simulink model "runTrajectoryFuzzy"  (R2019a)
settings: Solver=ode3  StartTime=0.0  StopTime=100.0  FixedStep=Ts  RelTol=1e-3
undefined symbols (not defined in the file): DiscIntNeverNeededParam, sigbuilder_block, th_0, Ts, x_0, y_0
libraries: simulink x3, fuzblock x1
settings Model: Creator=alvar  LastModifiedBy=alvar

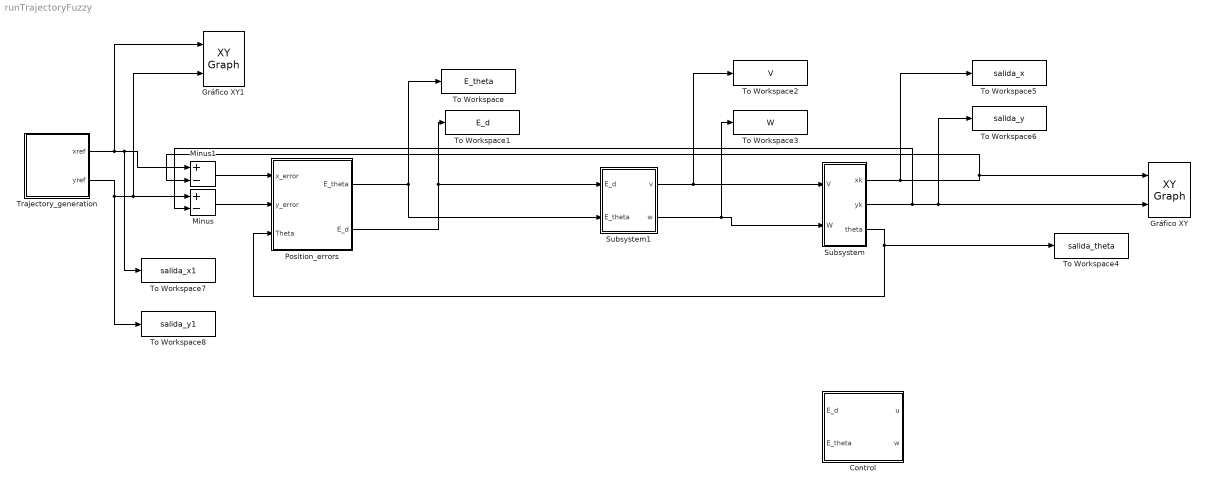
== system runTrajectoryFuzzy ==
  Control : Subsystem
  Gráfico XY : simulink/Sinks/XY Graph  xmin=-5  xmax=5  ymin=-5  ymax=5  st=-1
  Gráfico XY1 : simulink/Sinks/XY Graph  xmin=-5  xmax=5  ymin=-5  ymax=5  st=-1
  Minus : Sum  Inputs=+-
  Minus1 : Sum  Inputs=+-
  Position_errors : Subsystem
  Subsystem : Subsystem
  Subsystem1 : Subsystem
  To Workspace : ToWorkspace  VariableName=E_theta  SaveFormat=Structure With Time  SampleTime=-1
  To Workspace1 : ToWorkspace  VariableName=E_d  SaveFormat=Structure With Time  SampleTime=-1
  To Workspace2 : ToWorkspace  VariableName=V  SaveFormat=Structure With Time  SampleTime=-1
  To Workspace3 : ToWorkspace  VariableName=W  SaveFormat=Structure With Time  SampleTime=-1
  To Workspace4 : ToWorkspace  VariableName=salida_theta  SaveFormat=Structure With Time  SampleTime=-1
  To Workspace5 : ToWorkspace  VariableName=salida_x  SaveFormat=Structure With Time  SampleTime=-1
  To Workspace6 : ToWorkspace  VariableName=salida_y  SaveFormat=Structure With Time  SampleTime=-1
  To Workspace7 : ToWorkspace  VariableName=salida_x1  SaveFormat=Structure With Time  SampleTime=-1
  To Workspace8 : ToWorkspace  VariableName=salida_y1  SaveFormat=Structure With Time  SampleTime=-1
  Trajectory_generation : Subsystem
  wires:
  Position_errors/2(E_d) -> Subsystem1/1("E_d "), To Workspace1/1
  Subsystem1/1(v) -> To Workspace2/1, Subsystem/1(V)
  Minus/1 -> Position_errors/2("y_error ")
  Subsystem/1(xk) -> To Workspace5/1, Minus1/2, Gráfico XY/1
  Subsystem/3("theta ") -> Position_errors/3(Theta), To Workspace4/1
  Trajectory_generation/1(xref) -> Gráfico XY1/1, To Workspace7/1, Minus1/1
  Trajectory_generation/2(yref) -> To Workspace8/1, Gráfico XY1/2, Minus/1
  Subsystem/2(yk) -> Minus/2, To Workspace6/1, Gráfico XY/2
  Subsystem1/2(w) -> To Workspace3/1, Subsystem/2("W ")
  Position_errors/1(E_theta) -> Subsystem1/2(E_theta), To Workspace/1
  Minus1/1 -> Position_errors/1("x_error ")

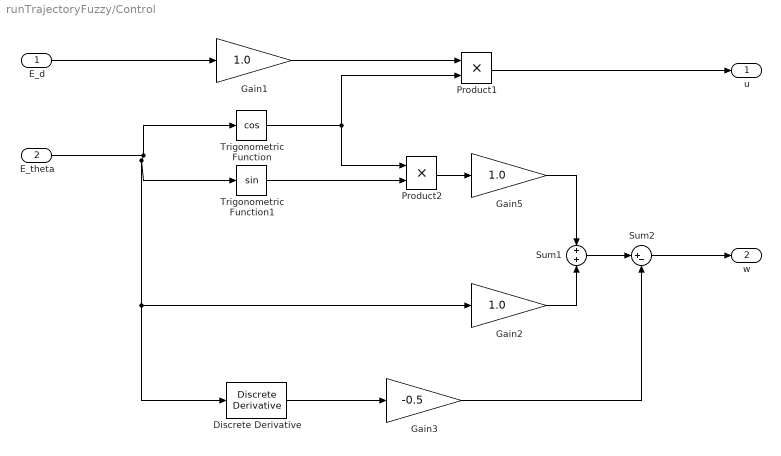
== system runTrajectoryFuzzy/Control ==
  E_d : Inport
  E_theta : Inport  Port=2
  Discrete Derivative : simulink/Discrete/Discrete Derivative  gainval=1.0  ICPrevScaledInput=0.0  OutMin=[]  OutMax=[]  OutDataType=fixdt(1, 16)  OutScaling=2^-10  DoSatur=off
  Gain1 : Gain  Gain=1.0
  Gain2 : Gain  Gain=1.0
  Gain3 : Gain  Gain=-0.5
  Gain5 : Gain  Gain=1.0
  Product1 : Product
  Product2 : Product
  Sum1 : Sum
  Sum2 : Sum  Inputs=|+-
  Trigonometric Function : Trigonometry  Operator=cos
  Trigonometric Function1 : Trigonometry
  u : Outport
  w : Outport  Port=2
  wires:
  E_theta/1 -> Trigonometric Function/1, Trigonometric Function1/1, Discrete Derivative/1, Gain2/1
  E_d/1 -> Gain1/1
  Trigonometric Function/1 -> Product1/2, Product2/1
  Trigonometric Function1/1 -> Product2/2
  Product2/1 -> Gain5/1
  Gain1/1 -> Product1/1
  Gain5/1 -> Sum1/1
  Gain2/1 -> Sum1/2
  Product1/1 -> u/1
  Sum1/1 -> Sum2/1
  Sum2/1 -> w/1
  Discrete Derivative/1 -> Gain3/1
  Gain3/1 -> Sum2/2

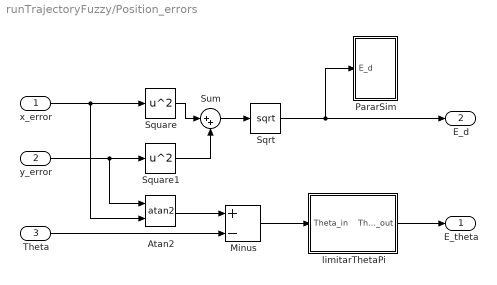
== system runTrajectoryFuzzy/Position_errors ==
  "x_error " : Inport
  "y_error " : Inport  Port=2
  Theta : Inport  Port=3
  Atan2 : Trigonometry  Operator=atan2
  Minus : Sum  Inputs=+-
  PararSim : Subsystem
  Sqrt : Sqrt  SaturateOnIntegerOverflow=on
  Square : Math  Operator=square  SaturateOnIntegerOverflow=on
  Square1 : Math  Operator=square  SaturateOnIntegerOverflow=on
  Sum : Sum  Inputs=|++
  limitarThetaPi : Subsystem
  E_theta : Outport  VectorParamsAs1DForOutWhenUnconnected=on
  E_d : Outport  Port=2  VectorParamsAs1DForOutWhenUnconnected=on
  wires:
  "x_error "/1 -> Square/1, Atan2/2
  "y_error "/1 -> Atan2/1, Square1/1
  Theta/1 -> Minus/2
  Sum/1 -> Sqrt/1
  Sqrt/1 -> PararSim/1("E_d "), E_d/1
  Square/1 -> Sum/1
  Square1/1 -> Sum/2
  Atan2/1 -> Minus/1
  Minus/1 -> limitarThetaPi/1(Theta_in)
  limitarThetaPi/1(Theta_out) -> E_theta/1

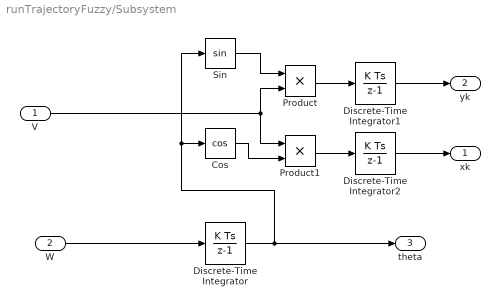
== system runTrajectoryFuzzy/Subsystem ==
  V : Inport
  "W " : Inport  Port=2
  Cos : Trigonometry  Operator=cos
  Discrete-Time Integrator : DiscreteIntegrator  InitialCondition=30*pi/180  SampleTime=-1  ICPrevOutput=DiscIntNeverNeededParam  ICPrevScaledInput=DiscIntNeverNeededParam
  Discrete-Time Integrator1 : DiscreteIntegrator  SampleTime=-1  ICPrevOutput=DiscIntNeverNeededParam  ICPrevScaledInput=DiscIntNeverNeededParam
  Discrete-Time Integrator2 : DiscreteIntegrator  SampleTime=-1  ICPrevOutput=DiscIntNeverNeededParam  ICPrevScaledInput=DiscIntNeverNeededParam
  Product : Product
  Product1 : Product
  Sin : Trigonometry
  xk : Outport  VectorParamsAs1DForOutWhenUnconnected=on
  yk : Outport  Port=2  VectorParamsAs1DForOutWhenUnconnected=on
  "theta " : Outport  Port=3  VectorParamsAs1DForOutWhenUnconnected=on
  wires:
  Discrete-Time Integrator2/1 -> xk/1
  Product/1 -> Discrete-Time Integrator1/1
  Cos/1 -> Product1/2
  Product1/1 -> Discrete-Time Integrator2/1
  Discrete-Time Integrator/1 -> "theta "/1, Sin/1, Cos/1
  V/1 -> Product1/1, Product/2
  "W "/1 -> Discrete-Time Integrator/1
  Discrete-Time Integrator1/1 -> yk/1
  Sin/1 -> Product/1

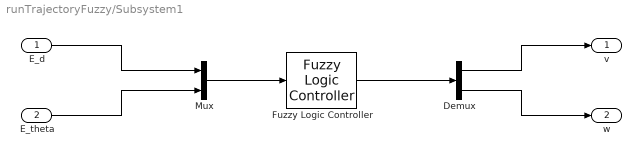
== system runTrajectoryFuzzy/Subsystem1 ==
  "E_d " : Inport
  E_theta : Inport  Port=2
  Demux : Demux  Outputs=2
  Fuzzy Logic Controller : fuzblock/Fuzzy Logic  Controller  FIS='practica2_g.fis'  OutputSampleNumber=101  DataType=double  FuzzifiedInputs=off  RuleFiringStrengths=off  RuleOutputs=off  AggregatedOutputs=off  SimulateUsing=Interpreted execution  OutOfRangeInputValueMessage=warning  NoRuleFiredMessage=warning  EmptyOutputFuzzySetMessage=warning
  Mux : Mux  Inputs=2
  v : Outport
  w : Outport  Port=2
  wires:
  Mux/1 -> Fuzzy Logic Controller/1
  Demux/1 -> v/1
  "E_d "/1 -> Mux/1
  E_theta/1 -> Mux/2
  Demux/2 -> w/1
  Fuzzy Logic Controller/1 -> Demux/1

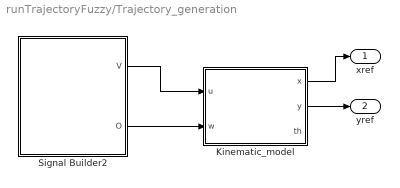
== system runTrajectoryFuzzy/Trajectory_generation ==
  Kinematic_model : Subsystem
  Signal Builder2 : Subsystem  Tag=STV Subsys  LoadFcn=sigbuilder_block('load');  StartFcn=sigbuilder_block('start');  StopFcn=sigbuilder_block('stop');  ClipboardFcn=sigbuilder_block('clipboard');  mask(Sigbuilder block){tuvar=[0:10]}
      mask help: Sigbuilder GUI
      mask init:
      | if ~strcmp(get_param(bdroot(gcbh),'SimulationStatus'),'stopped') tuvar = sigbuilder_block('maskInit'); end
      settings: CopyFcn=sigbuilder_block('copy');  DeleteFcn=sigbuilder_block('delete');  ModelCloseFcn=sigbuilder_block('modelClose');  PreSaveFcn=sigbuilder_block('preSave');  PauseFcn=sigbuilder_block('pause')  ContinueFcn=sigbuilder_block('continue')  NameChangeFcn=sigbuilder_block('namechange');  OpenFcn=sigbuilder_block('open',[60 82.4 534.4 508 ]);  CloseFcn=sigbuilder_block('close');
      mask Display: plot(0, 0, 100, 100,[2, 2, 32, 32, 2], [68, 8, 8, 68, 68],[32, 2], [38, 38], [32, 19, 2],[53, 60, 44], [32, 17, 17, 2],[16, 16, 31, 31]);txt = getActiveGroup(gcbh);text(2, 100, txt,'verticalAlignment', 'top');
  xref : Outport
  yref : Outport  Port=2
  wires:
  Signal Builder2/1(V) -> Kinematic_model/1(u)
  Signal Builder2/2(O) -> Kinematic_model/2(w)
  Kinematic_model/1(x) -> xref/1
  Kinematic_model/2(y) -> yref/1

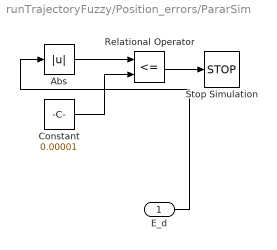
== system runTrajectoryFuzzy/Position_errors/PararSim ==
  "E_d " : Inport
  Abs : Abs
  Constant : Constant  Value=0.00001
  Relational Operator : RelationalOperator  Operator=<=  OutDataTypeStr=boolean  RndMeth=Simplest
  Stop Simulation : Stop
  wires:
  Abs/1 -> Relational Operator/1
  Constant/1 -> Relational Operator/2
  "E_d "/1 -> Abs/1
  Relational Operator/1 -> Stop Simulation/1

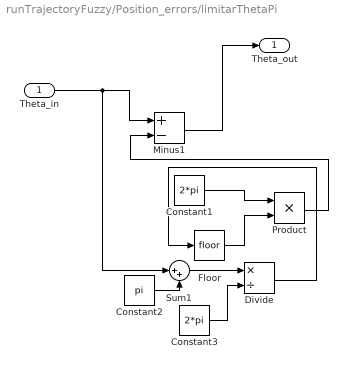
== system runTrajectoryFuzzy/Position_errors/limitarThetaPi ==
  Theta_in : Inport
  Constant1 : Constant  Value=2*pi
  Constant2 : Constant  Value=pi
  Constant3 : Constant  Value=2*pi
  Divide : Product  Inputs=*/
  Floor : Rounding
  Minus1 : Sum  Inputs=+-
  Product : Product
  Sum1 : Sum  Inputs=|++
  Theta_out : Outport
  wires:
  Constant1/1 -> Product/1
  Theta_in/1 -> Sum1/1, Minus1/1
  Sum1/1 -> Divide/1
  Floor/1 -> Product/2
  Minus1/1 -> Theta_out/1
  Constant2/1 -> Sum1/2
  Divide/1 -> Floor/1
  Product/1 -> Minus1/2
  Constant3/1 -> Divide/2

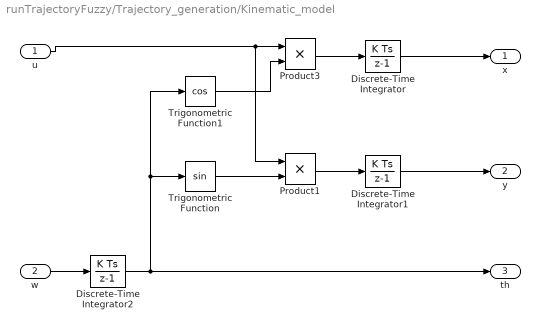
== system runTrajectoryFuzzy/Trajectory_generation/Kinematic_model ==
  u : Inport
  w : Inport  Port=2
  Discrete-Time Integrator : DiscreteIntegrator  InitialCondition=x_0  SampleTime=Ts  ICPrevOutput=DiscIntNeverNeededParam  ICPrevScaledInput=DiscIntNeverNeededParam
  Discrete-Time Integrator1 : DiscreteIntegrator  InitialCondition=y_0  SampleTime=Ts  ICPrevOutput=DiscIntNeverNeededParam  ICPrevScaledInput=DiscIntNeverNeededParam
  Discrete-Time Integrator2 : DiscreteIntegrator  InitialCondition=th_0  SampleTime=Ts  ICPrevOutput=DiscIntNeverNeededParam  ICPrevScaledInput=DiscIntNeverNeededParam
  Product1 : Product
  Product3 : Product
  Trigonometric Function : Trigonometry
  Trigonometric Function1 : Trigonometry  Operator=cos
  x : Outport
  y : Outport  Port=2
  th : Outport  Port=3
  wires:
  Discrete-Time Integrator2/1 -> Trigonometric Function1/1, Trigonometric Function/1, th/1
  Product1/1 -> Discrete-Time Integrator1/1
  Product3/1 -> Discrete-Time Integrator/1
  w/1 -> Discrete-Time Integrator2/1
  Trigonometric Function/1 -> Product1/2
  u/1 -> Product1/1, Product3/1
  Trigonometric Function1/1 -> Product3/2
  Discrete-Time Integrator1/1 -> y/1
  Discrete-Time Integrator/1 -> x/1

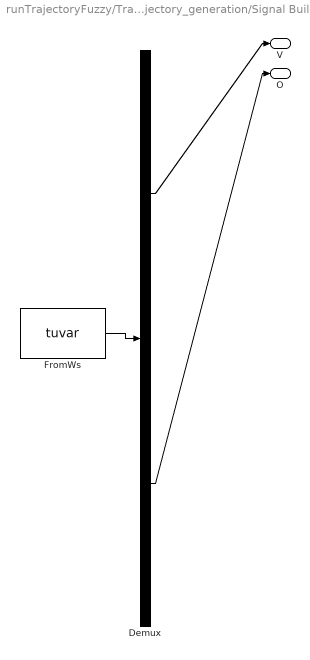
== system runTrajectoryFuzzy/Trajectory_generation/Signal Builder2 ==
  Demux : Demux  Tag=STV Demux  Outputs=2
  FromWs : FromWorkspace  Tag=STV FromWs  VariableName=tuvar  SampleTime=0
      SigBuilderData=|
      | common.afterFinalStr = 'Extrapolate'
      | common.sampleTime = '0'
      | dataSet.timeRange = [0 115]
      | dataSet.name = 'Group 1'
      | sbobj.Groups.Name = 'Group 1'
      | sbobj.Groups.Signals(1).Name = 'V'
      | sbobj.Groups.Signals(1).XData = [0 87 87 115]
      | sbobj.Groups.Signals(1).YData = [0.25 0.25 0 0]
      | sbobj.Groups.Signals(2).Name = 'O'
      | sbobj.Groups.Signals(2).XData = [0 12 12 30.849 30.849 55.981 55.981 74.83 74.83 99.962 115]
      | sbobj.Groups.Signals(2).YData = [0 0 0.25 0.25 -0.25 -0.25 0.25 0.25 0 0 0]
      | sbobj.Groups.TimeRange = [0 115]
  V : Outport  Tag=STV Outport
  O : Outport  Tag=STV Outport  Port=2
  wires:
  FromWs/1 -> Demux/1
  Demux/1 -> V/1
  Demux/2 -> O/1
